simulink library "icc_lib_avg_path1_n1"  (R2018b)
settings: Solver=VariableStepAuto  StartTime=0.0  StopTime=10.0  RelTol=1e-3
undefined symbols (not defined in the file or in its folder): icc_lib_avg_path, path1
libraries: simulink x34, simulink_extras x8, $bdroot x2
(part 3 of 4)

== matlab function icc_lib_avg_path1_n1/freqs ==
  data: cfg2 output; f input
function cfg2 = fcn(f)

% d0=-0.075;
% d1=43.625;
% d2=-0.88;
% d3=-8.65;


d0 = 0;
d1 = 43.5248;
d2= -0.909759259;
d3= -8.636136364;


% VT= -67.6336;
% Vm= -24.1075;
% VR= -28.8921;
% VF= -66.9586;

VT= -67.6339;
Vm= -24.1091;
VR= -28.9894;
VF= -66.9884;

switch f
    % 3.5 cpm
    case 17.15
%         d0 = -0.106346457;
%         d0 = -0.11255;
%         d0 = -0.11847;
        d0 = -0.116;

    % 3.2 cpm
    case 18.75
%         d0 = -0.084943396;
        d0 = -0.09004;
%         d0 = -0.093791667;

    case 20
        d0=-0.0767;
%         d0 = -0.073402174;
    case 20.05
        d0 = -0.073005405;
    case 20.1
       d0 = -0.072612903;
    case 20.15
       d0 = -0.072224599;
    case 20.2
       d0 = -0.071840426;
    case 20.25
       d0 = -0.071460317;
    case 20.3
       d0 = -0.071084211;
    case 20.35
       d0 = -0.070712042;
    case 20.4
       d0 = -0.07034375;
    case 20.45
       d0 = -0.069979275;
    case 20.5
       d0 = -0.069618557;
    case 20.55
       d0 = -0.069261538;
    case 20.6
       d0 = -0.068908163;
    case 20.65
       d0 = -0.068558376;
    case 20.7
       d0 = -0.068212121;
    case 20.75
       d0 = -0.067869347;
    case 20.8
       d0 = -0.06753;
    case 20.85
       d0 = -0.06719403;
    case 20.9
       d0 = -0.066861386;
    case 20.95
       d0 = -0.06653202;
    case 21
       d0 = -0.066205882;
    case 21.05
       d0 = -0.065882927;
    case 21.1
       d0 = -0.065563107;
    case 21.15
       d0 = -0.065246377;
    case 21.2
       d0 = -0.064932692;
    case 21.25
       d0 = -0.06462201;
    case 21.3
       d0 = -0.064314286;
    case 21.35
       d0 = -0.064009479;
    case 21.4
       d0 = -0.063707547;
    case 21.45
       d0 = -0.063408451;
    case 21.5
       d0 = -0.06311215;
    case 21.55
       d0 = -0.062818605;
    case 21.6
       d0 = -0.062527778;
    case 21.65
       d0 = -0.062239631;
    case 21.7
       d0 = -0.061954128;
    case 21.75
       d0 = -0.061671233;
    case 21.8
       d0 = -0.061390909;
    case 21.85
       d0 = -0.061113122;
    case 21.9
       d0 = -0.060837838;
    case 21.95
       d0 = -0.060565022;
    case 22
       d0 = -0.060294643;
    case 22.05
       d0 = -0.060026667;
    case 22.1
       d0 = -0.059761062;
    case 22.15
       d0 = -0.059497797;
    case 22.2
       d0 = -0.059236842;
    case 22.25
       d0 = -0.058978166;
    case 22.3
       d0 = -0.058721739;
    case 22.35
       d0 = -0.058467532;
    case 22.4
       d0 = -0.058215517;
    case 22.45
       d0 = -0.057965665;
    case 22.5
       d0 = -0.057717949;
    case 22.55
       d0 = -0.05747234;
    case 22.6
       d0 = -0.057228814;
    case 22.65
       d0 = -0.056987342;
    case 22.7
       d0 = -0.056747899;
    case 22.75
       d0 = -0.05651046;
    case 22.8
       d0 = -0.056275;
    case 22.85
       d0 = -0.056041494;
    case 22.9
       d0 = -0.055809917;
    case 22.95
       d0 = -0.055580247;
    case 23
       d0 = -0.055352459;
    case 23.05
       d0 = -0.055126531;
    case 23.1
       d0 = -0.054902439;
    case 23.15
       d0 = -0.054680162;
    case 23.2
       d0 = -0.054459677;
    case 23.25
       d0 = -0.054240964;
    case 23.3
       d0 = -0.054024;
    case 23.35
       d0 = -0.053808765;
    case 23.4
       d0 = -0.053595238;
    case 23.45
       d0 = -0.053383399;
    case 23.5
       d0 = -0.053173228;
    case 23.55
       d0 = -0.052964706;
    case 23.6
       d0 = -0.052757812;
    case 23.65
       d0 = -0.052552529;
    case 23.7
       d0 = -0.052348837;
    case 23.75
       d0 = -0.052146718;
    case 23.8
       d0 = -0.051946154;
    case 23.85
       d0 = -0.051747126;
    case 23.9
       d0 = -0.051549618;
    case 23.95
       d0 = -0.051353612;
    case 24
       d0 = -0.051159091;
    case 24.05
       d0 = -0.050966038;
    case 24.1
       d0 = -0.050774436;
    case 24.15
       d0 = -0.05058427;
    case 24.2
       d0 = -0.050395522;
    case 24.25
       d0 = -0.050208178;
    case 24.3
       d0 = -0.050022222;
    case 24.35
       d0 = -0.049837638;
    case 24.4
       d0 = -0.049654412;
    case 24.45
       d0 = -0.049472527;
    case 24.5
       d0 = -0.049291971;
    case 24.55
       d0 = -0.049112727;
    case 24.6
       d0 = -0.048934783;
    case 24.65
       d0 = -0.048758123;
    case 24.7
       d0 = -0.048582734;
    case 24.75
       d0 = -0.048408602;
    case 24.8
       d0 = -0.048235714;
    case 24.85
       d0 = -0.048064057;
    case 24.9
       d0 = -0.047893617;
    case 24.95
       d0 = -0.047724382;
    case 25
       d0 = -0.047556338;
    case 25.05
       d0 = -0.047389474;
    case 25.1
       d0 = -0.047223776;
    case 25.15
       d0 = -0.047059233;
    case 25.2
       d0 = -0.046895833;
    case 25.25
       d0 = -0.046733564;
    case 25.3
       d0 = -0.046572414;
    case 25.35
       d0 = -0.046412371;
    case 25.4
       d0 = -0.046253425;
    case 25.45
       d0 = -0.046095563;
    case 25.5
       d0 = -0.045938776;
    case 25.55
       d0 = -0.045783051;
    case 25.6
       d0 = -0.045628378;
    case 25.65
       d0 = -0.045474747;
    case 25.7
       d0 = -0.045322148;
    case 25.75
       d0 = -0.045170569;
    case 25.8
       d0 = -0.04502;
    case 25.85
       d0 = -0.044870432;
    case 25.9
       d0 = -0.044721854;
    case 25.95
       d0 = -0.044574257;
    case 26
       d0 = -0.044427632;

        
end


cfg2=[d0,d1,d2,d3,VT,Vm,VR,VF];

end

== stateflow chart icc_lib_avg_path1_n1/ICC1/Chart ==
  state wait
    entry:
    du:
    t2=temporalCount (sec);
  state q0
    en:
    q=0
  state q1
    en:
    q=1
    Sense=1;
    exit:
    Sense=0;
  state q3
    en:
    q=3
  state q2
    en:
    q=2
  (default) -> wait : {t2=0;}
  wait -> q0 : [t2>=19.6]{q=0;vreset=-67.6336;reset}
  q0 -> q1 [order 1] : [v<VT]/{vreset=v;Vmax=Vm;d2=d2i;reset}
  q0 -> q1 [order 2] : [gv>VF&&v>VT]{ vreset=gv; Vmax=Vm;d2=d2i;reset}
  q3 -> q0 : [v<VF]{vreset=v; reset}
  q1 -> q2 : [ v >Vmax ]{vreset=v; reset}
  q2 -> q3 : [v<VR]{vreset=v; reset}
  data: v input double; q output; vreset output; gv input double; VT input; Vm input; VR input; VF input; Vmax local; t2 local; d2i input; d2 output; Sense output
  events: reset output EITHER_EDGE_EVENT

== matlab function icc_lib_avg_path1_n1/ICC1/MATLAB Function ==
  data: cfg output
function cfg = fcn()

%d0-o= -0.039651515;
d0= -0.042051515;
d1= 216.5795;
d2= -0.7491129;
d3= -8.890176;
%d3-1= -8.960176;

VT= -67.6;
Vm= -24.3058;
VR= -28.9622;
VF= -66.9799;

cfg=[d0,d1,d2,d3,VT,Vm,VR,VF];

end

== matlab function icc_lib_avg_path1_n1/ICC1/MATLAB Function-freq=22  ==
  data: cfg2 output
function cfg2 = fcn()

%d0-o= -0.039651515;

%d0= -0.042051515;
%d1= 216.5795;
%d2= -0.7491129;
%d3= -8.890176;

%d3-1= -8.960176;

%freq=22
d0=-0.045;
d1=43.5373;
d2=-0.835;
d3=-6.96;


VT= -67.6336;
Vm= -24.1075;
VR= -28.8921;
VF= -66.9586;



cfg2=[d0,d1,d2,d3,VT,Vm,VR,VF];

end

== matlab function icc_lib_avg_path1_n1/freq20 ==
  data: cfg2 output
function cfg2 = fcn()

%d0-o= -0.039651515;

%d0= -0.042051515;
%d1= 216.5795;
%d2= -0.7491129;
%d3= -8.890176;

%d3-1= -8.960176;


d0=-0.075;
d1=43.625;
d2=-0.88;
d3=-8.65;


VT= -67.6336;
Vm= -24.1075;
VR= -28.8921;
VF= -66.9586;



cfg2=[d0,d1,d2,d3,VT,Vm,VR,VF];

end

== stateflow chart icc_lib_avg_path1_n1/Chart1 ==
  state q01
    du:
    t1=temporalCount (sec);
    pulse=-69;
  state q002
    en:m=0;
    du:
    t=temporalCount (sec);
    pulse=-67.6;
  state q001
    en:m=m+1;
    du:
    t=temporalCount (sec);
    pulse=-67.6;
  state state
    en: pulse = -67.6;
  state end
  (default) -> q002 : {m=0; t=0;}
  q001 -> q01 [order 1] : [ t >=5]{ t1=0;}
  q002 -> q001 : [t>=10]{t=0;}
  q01 -> q001 : [t1>=(0.8)]{t=0;}
  q001 -> state [order 2] : [m>6]
  state -> end
  data: m local; t local; t1 local; pulse output

== matlab function icc_lib_avg_path1_n1/ICC /MATLAB Function-freq=26  ==
  data: cfg2 output
function cfg2 = fcn()

%d0-o= -0.039651515;

%d0= -0.042051515;
%d1= 216.5795;
%d2= -0.7491129;
%d3= -8.890176;

%d3-1= -8.960176;

%freq26
d0=-0.053;
d1=39.5735;
d2=-0.8035;
d3=-4.69678;


VT= -67.6336;
Vm= -24.1075;
VR= -28.8921;
VF= -66.9586;



cfg2=[d0,d1,d2,d3,VT,Vm,VR,VF];

end

== stateflow chart icc_lib_avg_path1_n1/ICC-multi/Chart ==
  state wait
    entry:
    du:
    t2=temporalCount (sec);
  state q0
    en:
    q=0
  state q1
    en:
    q=1
  state q3
    en:
    q=3
  state q2
    en:
    q=2
  (default) -> wait : {t2=0;}
  wait -> q0 : [t2>=19.6]{q=0;th=0;vreset=-67.6;reset}
  q0 -> q1 [order 1] : [v<VT]/{vreset=v; th=0; Vmax=Vm;d2=d2i; reset}
  q0 -> q1 [order 2] : [gv>VF&&v>VT]{ vreset=v; th=v-VT/VF-VT; Vmax=func1(th,Vm);d2=func2(th,d2i);reset}
  q3 -> q0 : [v<VF]{vreset=-67; reset}
  q1 -> q2 : [ v >Vmax ]{vreset=v; reset}
  q2 -> q3 : [v<VR]{vreset=v; reset}
  data: vmax function_output double; theta function_input; vm function_input; d2out function_output double; theta function_input; d2in function_input; v input double; q output; vreset output; gv input double; Vmm input; VT input; Vm input; VR input; VF input; th local; Vmax local; t2 local; d2i input; d2 output
  events: reset output EITHER_EDGE_EVENT
  function vmax = func1(theta,vm):
    | function vmax = func1(theta,vm)
    | 
    | m=1;
    | 
    | 
    | vmax1=Vm*exp(-m*th);
    | vmax=-25
  function d2out = func2(theta,d2in):
    | function d2out = func2(theta,d2in)
    | 
    | m=1;
    | 
    | 
    | vmax1=Vm*exp(-m*th);
    | %d2out=-0.5
    | d2out=d2in;

== stateflow chart icc_lib_avg_path1_n1/path/Path ==
  state Relay_cell1
  state Relay_cell2
  state Previous_Direction1
  state Idle
  state Previous_Direction2
  state Wait_cell2
  state Wait_cell1
  state Annihilate
  Wait_cell1 -> Relay_cell1 [order 2] : after(0.1, sec) /
      | {relay1 = 1;
      | last = 1;}
  Wait_cell2 -> Relay_cell2 [order 2] : after(0.1, sec) /
      | {relay2 = 1;
      | last = 2;}
  Relay_cell1 -> Idle : after(0.1, sec) /
      | {relay1 = 0;}
  Relay_cell2 -> Idle : after(0.1, sec) /
      | {relay2 = 0;}
  (default) -> Idle
  Idle -> Previous_Direction2 [order 3] : [mode2 == 2 ...
      | && mode1 ~= 2]
  Previous_Direction2 -> Wait_cell2 [order 2] : [last == 0]
  Idle -> Previous_Direction1 [order 2] : [mode1 == 2 ...
      | && mode2 ~= 2]
  Previous_Direction1 -> Wait_cell1 [order 2] : [last == 0]
  Idle -> Annihilate [order 1] : [mode1 == 2 ...
      | && mode2 == 2]
  Annihilate -> Idle : [mode1 ~= 2 ...
      | && mode2 ~= 2] /
      | {last = 0;}
  Previous_Direction2 -> Wait_cell2 [order 3] : [last == 2]
  Previous_Direction1 -> Wait_cell1 [order 3] : [last == 1]
  Previous_Direction2 -> Wait_cell2 [order 4] : [last == 1 && ...
      | mdelay1 == 0]
  Previous_Direction1 -> Wait_cell1 [order 4] : [last == 2 && ...
      | mdelay2 == 0]
  Wait_cell2 -> Annihilate [order 1] : [mode1 == 2]
  Wait_cell1 -> Annihilate [order 1] : [mode2 == 2]
  Previous_Direction1 -> Annihilate [order 1] : [last == 2 && ...
      | mdelay2 ~= 0]
  Previous_Direction2 -> Annihilate [order 1] : [last == 1 && ...
      | mdelay1 ~= 0]
  data: mode1 input; mdelay1 input; mode2 input; mdelay2 input; relay1 output; relay2 output; last local; cell1_mode_delayed local; cell2_mode_delayed local

== matlab function icc_lib_avg_path1_n1/ICC-multi/MATLAB Function ==
  data: cfg output
function cfg = fcn()

%d0-o= -0.039651515;
d0= -0.042051515;
d1= 216.5795;
d2= -0.7491129;
d3= -8.890176;
%d3-1= -8.960176;

VT= -67.6;
Vm= -24.3058;
VR= -28.9622;
VF= -66.9799;

cfg=[d0,d1,d2,d3,VT,Vm,VR,VF];

end

== matlab function icc_lib_avg_path1_n1/ICC-multi/MATLAB Function-freq=22  ==
  data: cfg2 output
function cfg2 = fcn()

%d0-o= -0.039651515;

%d0= -0.042051515;
%d1= 216.5795;
%d2= -0.7491129;
%d3= -8.890176;

%d3-1= -8.960176;

%freq=22
d0=-0.045;
d1=43.5373;
d2=-0.835;
d3=-6.96;


VT= -67.6336;
Vm= -24.1075;
VR= -28.8921;
VF= -66.9586;



cfg2=[d0,d1,d2,d3,VT,Vm,VR,VF];

end

== matlab function icc_lib_avg_path1_n1/ICC-multi/MATLAB Function-freq=24 ==
  data: cfg2 output
function cfg2 = fcn()

%d0-o= -0.039651515;

%d0= -0.042051515;
%d1= 216.5795;
%d2= -0.7491129;
%d3= -8.890176;

%d3-1= -8.960176;

%freq24
d0=-0.0381;
d1=43.568;
d2=-0.82;
d3=-4.8;


VT= -67.6336;
Vm= -24.1075;
VR= -28.8921;
VF= -66.9586;



cfg2=[d0,d1,d2,d3,VT,Vm,VR,VF];

end

== matlab function icc_lib_avg_path1_n1/ICC-multi/MATLAB Function-freq=26  ==
  data: cfg2 output
function cfg2 = fcn()

%d0-o= -0.039651515;

%d0= -0.042051515;
%d1= 216.5795;
%d2= -0.7491129;
%d3= -8.890176;

%d3-1= -8.960176;

%freq26
d0=-0.053;
d1=39.5735;
d2=-0.8035;
d3=-4.69678;


VT= -67.6336;
Vm= -24.1075;
VR= -28.8921;
VF= -66.9586;



cfg2=[d0,d1,d2,d3,VT,Vm,VR,VF];

end

== matlab function icc_lib_avg_path1_n1/ICC-multi/MATLAB Function-freq=26-o  ==
  data: cfg2 output
function cfg2 = fcn()

%d0-o= -0.039651515;

%d0= -0.042051515;
%d1= 216.5795;
%d2= -0.7491129;
%d3= -8.890176;

%d3-1= -8.960176;

%freq26
d0=-0.053;
d1=39.5735;
d2=-0.8035;
d3=-4.69678;


VT= -67.6336;
Vm= -24.1075;
VR= -28.8921;
VF= -66.9586;



cfg2=[d0,d1,d2,d3,VT,Vm,VR,VF];

end

== matlab function icc_lib_avg_path1_n1/ICC-multi/MATLAB Function1-freq=20  ==
  data: cfg2 output
function cfg2 = fcn()

%d0-o= -0.039651515;

%d0= -0.042051515;
%d1= 216.5795;
%d2= -0.7491129;
%d3= -8.890176;

%d3-1= -8.960176;


d0=-0.075;
d1=43.625;
d2=-0.88;
d3=-8.65;


VT= -67.6336;
Vm= -24.1075;
VR= -28.8921;
VF= -66.9586;



cfg2=[d0,d1,d2,d3,VT,Vm,VR,VF];

end

== matlab function icc_lib_avg_path1_n1/ICC1/MATLAB Function-freq=24 ==
  data: cfg2 output
function cfg2 = fcn()

%d0-o= -0.039651515;

%d0= -0.042051515;
%d1= 216.5795;
%d2= -0.7491129;
%d3= -8.890176;

%d3-1= -8.960176;

%freq24
d0=-0.0381;
d1=43.568;
d2=-0.82;
d3=-4.8;


VT= -67.6336;
Vm= -24.1075;
VR= -28.8921;
VF= -66.9586;



cfg2=[d0,d1,d2,d3,VT,Vm,VR,VF];

end

== matlab function icc_lib_avg_path1_n1/ICC1/MATLAB Function-freq=26  ==
  data: cfg2 output
function cfg2 = fcn()

%d0-o= -0.039651515;

%d0= -0.042051515;
%d1= 216.5795;
%d2= -0.7491129;
%d3= -8.890176;

%d3-1= -8.960176;

%freq26
d0=-0.053;
d1=39.5735;
d2=-0.8035;
d3=-4.69678;


VT= -67.6336;
Vm= -24.1075;
VR= -28.8921;
VF= -66.9586;



cfg2=[d0,d1,d2,d3,VT,Vm,VR,VF];

end

== matlab function icc_lib_avg_path1_n1/ICC1/MATLAB Function-freq=26-o  ==
  data: cfg2 output
function cfg2 = fcn()

%d0-o= -0.039651515;

%d0= -0.042051515;
%d1= 216.5795;
%d2= -0.7491129;
%d3= -8.890176;

%d3-1= -8.960176;

%freq26
d0=-0.053;
d1=39.5735;
d2=-0.8035;
d3=-4.69678;


VT= -67.6336;
Vm= -24.1075;
VR= -28.8921;
VF= -66.9586;



cfg2=[d0,d1,d2,d3,VT,Vm,VR,VF];

end

== matlab function icc_lib_avg_path1_n1/ICC1/MATLAB Function1-freq=20  ==
  data: cfg2 output
function cfg2 = fcn()

%d0-o= -0.039651515;

%d0= -0.042051515;
%d1= 216.5795;
%d2= -0.7491129;
%d3= -8.890176;

%d3-1= -8.960176;


d0=-0.075;
d1=43.625;
d2=-0.88;
d3=-8.65;


VT= -67.6336;
Vm= -24.1075;
VR= -28.8921;
VF= -66.9586;



cfg2=[d0,d1,d2,d3,VT,Vm,VR,VF];

end

== stateflow chart icc_lib_avg_path1_n1/ICC6/Chart ==
  state block
    en:
    q=4
  state wait
    entry:
    du:
    t2=temporalCount (sec);
  state q0
    en:
    q=0
  state q1
    en:
    q=1
    Sense=1
    exit:
    Sense=0
  state q3
    en:
    q=3
  state q2
    en:
    q=2
  wait -> (junction 82) : [t2>=19.6]{q=0;th=0;vreset=-67.6336;reset}
  (junction 82) -> block [order 2] : [b==1]
  (junction 82) -> q0 [order 1] : [b==0]
  (default) -> wait : {t2=0;}
  q0 -> block [order 3] : [b==1]
  block -> q0 : [b==0]
  q0 -> q1 [order 1] : [v<VT]/{vreset=v; th=0; Vmax=Vm;d2=d2i; reset}
  q0 -> q1 [order 2] : [gv>VF&&v>VT]{ vreset=gv; th=v-VT/VF-VT; Vmax=func1(th,Vm);d2=func2(th,d2i);reset}
  q3 -> q0 : [v<VF]{vreset=v; reset}
  q1 -> q2 : [ v >Vmax ]{vreset=v; reset}
  q2 -> q3 : [v<VR]{vreset=v; reset}
  data: vmax function_output double; theta function_input; vm function_input; d2out function_output double; theta function_input; d2in function_input; v input double; q output; vreset output; gv input double; Vmm input; VT input; Vm input; VR input; VF input; th local; Vmax local; t2 local; d2i input; d2 output; b input; Sense output
  events: reset output EITHER_EDGE_EVENT
  function vmax = func1(theta,vm):
    | function vmax = func1(theta,vm)
    | 
    | m=1;
    | 
    | 
    | vmax1=Vm*exp(-m*th);
    | vmax=-25
  function d2out = func2(theta,d2in):
    | function d2out = func2(theta,d2in)
    | 
    | m=1;
    | 
    | 
    | vmax1=Vm*exp(-m*th);
    | %d2out=-0.5
    | d2out=d2in;

== matlab function icc_lib_avg_path1_n1/ICC6/MATLAB Function ==
  data: cfg output
function cfg = fcn()

%d0-o= -0.039651515;
d0= -0.042051515;
d1= 216.5795;
d2= -0.7491129;
d3= -8.890176;
%d3-1= -8.960176;

VT= -67.6;
Vm= -24.3058;
VR= -28.9622;
VF= -66.9799;

cfg=[d0,d1,d2,d3,VT,Vm,VR,VF];

end

== matlab function icc_lib_avg_path1_n1/ICC6/MATLAB Function-freq=22  ==
  data: cfg2 output
function cfg2 = fcn()

%d0-o= -0.039651515;

%d0= -0.042051515;
%d1= 216.5795;
%d2= -0.7491129;
%d3= -8.890176;

%d3-1= -8.960176;

%freq=22
d0=-0.045;
d1=43.5373;
d2=-0.835;
d3=-6.96;


VT= -67.6336;
Vm= -24.1075;
VR= -28.8921;
VF= -66.9586;



cfg2=[d0,d1,d2,d3,VT,Vm,VR,VF];

end

== matlab function icc_lib_avg_path1_n1/ICC6/MATLAB Function-freq=24 ==
  data: cfg2 output
function cfg2 = fcn()

%d0-o= -0.039651515;

%d0= -0.042051515;
%d1= 216.5795;
%d2= -0.7491129;
%d3= -8.890176;

%d3-1= -8.960176;

%freq24
d0=-0.0381;
d1=43.568;
d2=-0.82;
d3=-4.8;


VT= -67.6336;
Vm= -24.1075;
VR= -28.8921;
VF= -66.9586;



cfg2=[d0,d1,d2,d3,VT,Vm,VR,VF];

end

== matlab function icc_lib_avg_path1_n1/ICC6/MATLAB Function-freq=26  ==
  data: cfg2 output
function cfg2 = fcn()

%d0-o= -0.039651515;

%d0= -0.042051515;
%d1= 216.5795;
%d2= -0.7491129;
%d3= -8.890176;

%d3-1= -8.960176;

%freq26
d0=-0.053;
d1=39.5735;
d2=-0.8035;
d3=-4.69678;


VT= -67.6336;
Vm= -24.1075;
VR= -28.8921;
VF= -66.9586;



cfg2=[d0,d1,d2,d3,VT,Vm,VR,VF];

end

== matlab function icc_lib_avg_path1_n1/ICC6/MATLAB Function-freq=26-o  ==
  data: cfg2 output
function cfg2 = fcn()

%d0-o= -0.039651515;

%d0= -0.042051515;
%d1= 216.5795;
%d2= -0.7491129;
%d3= -8.890176;

%d3-1= -8.960176;

%freq26
d0=-0.053;
d1=39.5735;
d2=-0.8035;
d3=-4.69678;


VT= -67.6336;
Vm= -24.1075;
VR= -28.8921;
VF= -66.9586;



cfg2=[d0,d1,d2,d3,VT,Vm,VR,VF];

end

== matlab function icc_lib_avg_path1_n1/ICC6/MATLAB Function1-freq=20  ==
  data: cfg2 output
function cfg2 = fcn()

%d0-o= -0.039651515;

%d0= -0.042051515;
%d1= 216.5795;
%d2= -0.7491129;
%d3= -8.890176;

%d3-1= -8.960176;


d0=-0.075;
d1=43.625;
d2=-0.88;
d3=-8.65;


VT= -67.6336;
Vm= -24.1075;
VR= -28.8921;
VF= -66.9586;



cfg2=[d0,d1,d2,d3,VT,Vm,VR,VF];

end

== stateflow chart icc_lib_avg_path1_n1/ICC5/Chart ==
  state block
    en:
    q=4
  state wait
    entry:
    du:
    t2=temporalCount (sec);
  state q0
    en:
    q=0
  state q1
    en:
    q=1
    Sense=1
    exit:
    Sense=0
  state q3
    en:
    q=3
  state q2
    en:
    q=2
  wait -> (junction 82) : [t2>=19.6]{q=0;th=0;vreset=-67.6336;reset}
  (junction 82) -> block [order 2] : [b==1]
  (junction 82) -> q0 [order 1] : [b==0]
  (default) -> wait : {t2=0;}
  q0 -> block [order 3] : [b==1]
  block -> q0 : [b==0]
  q0 -> q1 [order 1] : [v<VT]/{vreset=v; th=0; Vmax=Vm;d2=d2i; reset}
  q0 -> q1 [order 2] : [gv>VF&&v>VT]{ vreset=gv; th=v-VT/VF-VT; Vmax=func1(th,Vm);d2=func2(th,d2i);reset}
  q3 -> q0 : [v<VF]{vreset=v; reset}
  q1 -> q2 : [ v >Vmax ]{vreset=v; reset}
  q2 -> q3 : [v<VR]{vreset=v; reset}
  data: vmax function_output double; theta function_input; vm function_input; d2out function_output double; theta function_input; d2in function_input; v input double; q output; vreset output; gv input double; Vmm input; VT input; Vm input; VR input; VF input; th local; Vmax local; t2 local; d2i input; d2 output; b input; Sense output
  events: reset output EITHER_EDGE_EVENT
  function vmax = func1(theta,vm):
    | function vmax = func1(theta,vm)
    | 
    | m=1;
    | 
    | 
    | vmax1=Vm*exp(-m*th);
    | vmax=-25
  function d2out = func2(theta,d2in):
    | function d2out = func2(theta,d2in)
    | 
    | m=1;
    | 
    | 
    | vmax1=Vm*exp(-m*th);
    | %d2out=-0.5
    | d2out=d2in;

== matlab function icc_lib_avg_path1_n1/ICC5/MATLAB Function ==
  data: cfg output
function cfg = fcn()

%d0-o= -0.039651515;
d0= -0.042051515;
d1= 216.5795;
d2= -0.7491129;
d3= -8.890176;
%d3-1= -8.960176;

VT= -67.6;
Vm= -24.3058;
VR= -28.9622;
VF= -66.9799;

cfg=[d0,d1,d2,d3,VT,Vm,VR,VF];

end

== matlab function icc_lib_avg_path1_n1/ICC5/MATLAB Function-freq=22  ==
  data: cfg2 output
function cfg2 = fcn()

%d0-o= -0.039651515;

%d0= -0.042051515;
%d1= 216.5795;
%d2= -0.7491129;
%d3= -8.890176;

%d3-1= -8.960176;

%freq=22
d0=-0.045;
d1=43.5373;
d2=-0.835;
d3=-6.96;


VT= -67.6336;
Vm= -24.1075;
VR= -28.8921;
VF= -66.9586;



cfg2=[d0,d1,d2,d3,VT,Vm,VR,VF];

end

== matlab function icc_lib_avg_path1_n1/ICC5/MATLAB Function-freq=24 ==
  data: cfg2 output
function cfg2 = fcn()

%d0-o= -0.039651515;

%d0= -0.042051515;
%d1= 216.5795;
%d2= -0.7491129;
%d3= -8.890176;

%d3-1= -8.960176;

%freq24
d0=-0.0381;
d1=43.568;
d2=-0.82;
d3=-4.8;


VT= -67.6336;
Vm= -24.1075;
VR= -28.8921;
VF= -66.9586;



cfg2=[d0,d1,d2,d3,VT,Vm,VR,VF];

end

== matlab function icc_lib_avg_path1_n1/ICC5/MATLAB Function-freq=26  ==
  data: cfg2 output
function cfg2 = fcn()

%d0-o= -0.039651515;

%d0= -0.042051515;
%d1= 216.5795;
%d2= -0.7491129;
%d3= -8.890176;

%d3-1= -8.960176;

%freq26
d0=-0.053;
d1=39.5735;
d2=-0.8035;
d3=-4.69678;


VT= -67.6336;
Vm= -24.1075;
VR= -28.8921;
VF= -66.9586;



cfg2=[d0,d1,d2,d3,VT,Vm,VR,VF];

end

== matlab function icc_lib_avg_path1_n1/ICC5/MATLAB Function-freq=26-o  ==
  data: cfg2 output
function cfg2 = fcn()

%d0-o= -0.039651515;

%d0= -0.042051515;
%d1= 216.5795;
%d2= -0.7491129;
%d3= -8.890176;

%d3-1= -8.960176;

%freq26
d0=-0.053;
d1=39.5735;
d2=-0.8035;
d3=-4.69678;


VT= -67.6336;
Vm= -24.1075;
VR= -28.8921;
VF= -66.9586;



cfg2=[d0,d1,d2,d3,VT,Vm,VR,VF];

end

== matlab function icc_lib_avg_path1_n1/ICC5/MATLAB Function1-freq=20  ==
  data: cfg2 output
function cfg2 = fcn()

%d0-o= -0.039651515;

%d0= -0.042051515;
%d1= 216.5795;
%d2= -0.7491129;
%d3= -8.890176;

%d3-1= -8.960176;


d0=-0.075;
d1=43.625;
d2=-0.88;
d3=-8.65;


VT= -67.6336;
Vm= -24.1075;
VR= -28.8921;
VF= -66.9586;



cfg2=[d0,d1,d2,d3,VT,Vm,VR,VF];

end

== stateflow chart icc_lib_avg_path1_n1/ICC7/Chart ==
  state block
    en:
    q=4
  state wait
    entry:
    du:
    t2=temporalCount (sec);
  state q0
    en:
    q=0
  state q1
    en:
    q=1
    Sense=1
    exit:
    Sense=0
  state q3
    en:
    q=3
  state q2
    en:
    q=2
  wait -> (junction 82) : [t2>=19.6]{q=0;th=0;vreset=-67.6336;reset}
  (junction 82) -> block [order 2] : [b==1]
  (junction 82) -> q0 [order 1] : [b==0]
  (default) -> wait : {t2=0;}
  q0 -> block [order 3] : [b==1]
  block -> q0 : [b==0]
  q0 -> q1 [order 1] : [v<VT]/{vreset=v; th=0; Vmax=Vm;d2=d2i; reset}
  q0 -> q1 [order 2] : [gv>VF&&v>VT]{ vreset=gv; th=v-VT/VF-VT; Vmax=func1(th,Vm);d2=func2(th,d2i);reset}
  q3 -> q0 : [v<VF]{vreset=v; reset}
  q1 -> q2 : [ v >Vmax ]{vreset=v; reset}
  q2 -> q3 : [v<VR]{vreset=v; reset}
  data: vmax function_output double; theta function_input; vm function_input; d2out function_output double; theta function_input; d2in function_input; v input double; q output; vreset output; gv input double; Vmm input; VT input; Vm input; VR input; VF input; th local; Vmax local; t2 local; d2i input; d2 output; b input; Sense output
  events: reset output EITHER_EDGE_EVENT
  function vmax = func1(theta,vm):
    | function vmax = func1(theta,vm)
    | 
    | m=1;
    | 
    | 
    | vmax1=Vm*exp(-m*th);
    | vmax=-25
  function d2out = func2(theta,d2in):
    | function d2out = func2(theta,d2in)
    | 
    | m=1;
    | 
    | 
    | vmax1=Vm*exp(-m*th);
    | %d2out=-0.5
    | d2out=d2in;

== matlab function icc_lib_avg_path1_n1/ICC7/MATLAB Function ==
  data: cfg output
function cfg = fcn()

%d0-o= -0.039651515;
d0= -0.042051515;
d1= 216.5795;
d2= -0.7491129;
d3= -8.890176;
%d3-1= -8.960176;

VT= -67.6;
Vm= -24.3058;
VR= -28.9622;
VF= -66.9799;

cfg=[d0,d1,d2,d3,VT,Vm,VR,VF];

end

== matlab function icc_lib_avg_path1_n1/ICC7/MATLAB Function-freq=22  ==
  data: cfg2 output
function cfg2 = fcn()

%d0-o= -0.039651515;

%d0= -0.042051515;
%d1= 216.5795;
%d2= -0.7491129;
%d3= -8.890176;

%d3-1= -8.960176;

%freq=22
d0=-0.045;
d1=43.5373;
d2=-0.835;
d3=-6.96;


VT= -67.6336;
Vm= -24.1075;
VR= -28.8921;
VF= -66.9586;



cfg2=[d0,d1,d2,d3,VT,Vm,VR,VF];

end

== stateflow chart icc_lib_avg_path1_n1/Subsystem/Chart ==
  state Pacemaker
    state GRP [parallel]
      settings: executionOrder=1
      state Idle
        du:
        sense=Sense;
      state StartGRP
        du:
        grp=1;
        Tgrp=temporalCount (sec);
      state EndGRP
        en:
        grp=0;
        endGRP=1;
      state Wait
      (default) -> Pacemaker.GRP.Idle : {grp=0;Tgrp=0;endGRP=0;sense=0;}
      Pacemaker.GRP.Idle -> StartGRP [order 1] : [sense==1&&grp==0]{sense=0;}
      StartGRP -> EndGRP : [Tgrp==5]{Tgrp=0;}
      Pacemaker.GRP.Idle -> Pacemaker.GRP.Wait [order 2] : [sense==1&&grp==1]{sense=0;}
      EndGRP -> Pacemaker.GRP.Idle
      Pacemaker.GRP.Wait -> Pacemaker.GRP.Idle
    state LRI [parallel]
      settings: executionOrder=2
      state StartLRI
        en:
        c = c +1;
        du:
        Tlri=temporalCount (sec);
      state EndLRI
        en:
        pace=2;
        du:
        s=Sense
      state Idle
        du:
        s=Sense;
      state wait
      state Wait
      state AfterGRPsense
      (default) -> Pacemaker.LRI.Idle : {Tlri=0;grp=0;endGRP=0;s=0;c=0;}
      StartLRI -> EndLRI [order 1] : [Tlri>func3(c)&&sense==0]{Tlri=0}
      Pacemaker.LRI.Idle -> StartLRI [order 1] : [s==1&&grp==0]{s=0;}
      EndLRI -> StartLRI : [s==1]{pace=0;s=0;endGRP=0}
      Pacemaker.LRI.Wait -> Pacemaker.LRI.Idle
      Pacemaker.LRI.Idle -> Pacemaker.LRI.Wait [order 2] : [s==1&&grp==1]{s=0;}
      AfterGRPsense -> StartLRI
      StartLRI -> AfterGRPsense [order 3] : [endGRP==1&&Tlri<=func3(c)&&sense==1]{Tlri=0;endGRP=0;s=0}
      wait -> StartLRI
      StartLRI -> wait [order 2] : [endGRP==0&&Tlri<=func3(c)&&sense==1]{s=0;}
  (default) -> Pacemaker : {pace=0;}
  data: s local; c local; tlri function_output double; count function_input; pace output; Sense input; Tgrp local; Tlri local; grp local; endGRP local; sense local
  function tlri = func3(count):
    | function tlri = func3(count)
    | 
    | % LRI=19.9;
    | % offset=0.6;
    | 
    | % LRI=19.9-0.2-0.2+0.1;
    | 
    | %pace at s20
    | % offset=0.6+1.6+0.2-0.4;
    | 
    | % pace at s0 (sense and pace at every 20ns, (reveive pace and go upstroke at20n.1s)
    | % LRI = 19.6 making the fixed period as 20s, pace at what expected time use offeset 
    | LRI=19.9-0.2-0.2+0.1; %(LRI = 19.6)
    | offset=0.6+0.2-0.6-0.1; %(offset = 0.1)
    | 
    | % one second delay, i.e.if go upstroke at 20ns, then sense and pace one step advance,i.e set offset as 0 
    | 
    | 
    | %tlri=0;
    | if(count==1)
    |   tlri = LRI+offset;
    | 
    | %elseif(count>1)
    | else
    |   tlri = LRI;
    | 
    | end

== matlab function icc_lib_avg_path1_n1/ICC7/MATLAB Function-freq=24 ==
  data: cfg2 output
function cfg2 = fcn()

%d0-o= -0.039651515;

%d0= -0.042051515;
%d1= 216.5795;
%d2= -0.7491129;
%d3= -8.890176;

%d3-1= -8.960176;

%freq24
d0=-0.0381;
d1=43.568;
d2=-0.82;
d3=-4.8;


VT= -67.6336;
Vm= -24.1075;
VR= -28.8921;
VF= -66.9586;



cfg2=[d0,d1,d2,d3,VT,Vm,VR,VF];

end

== matlab function icc_lib_avg_path1_n1/ICC7/MATLAB Function-freq=26  ==
  data: cfg2 output
function cfg2 = fcn()

%d0-o= -0.039651515;

%d0= -0.042051515;
%d1= 216.5795;
%d2= -0.7491129;
%d3= -8.890176;

%d3-1= -8.960176;

%freq26
d0=-0.053;
d1=39.5735;
d2=-0.8035;
d3=-4.69678;


VT= -67.6336;
Vm= -24.1075;
VR= -28.8921;
VF= -66.9586;



cfg2=[d0,d1,d2,d3,VT,Vm,VR,VF];

end

== matlab function icc_lib_avg_path1_n1/ICC7/MATLAB Function-freq=26-o  ==
  data: cfg2 output
function cfg2 = fcn()

%d0-o= -0.039651515;

%d0= -0.042051515;
%d1= 216.5795;
%d2= -0.7491129;
%d3= -8.890176;

%d3-1= -8.960176;

%freq26
d0=-0.053;
d1=39.5735;
d2=-0.8035;
d3=-4.69678;


VT= -67.6336;
Vm= -24.1075;
VR= -28.8921;
VF= -66.9586;



cfg2=[d0,d1,d2,d3,VT,Vm,VR,VF];

end

== matlab function icc_lib_avg_path1_n1/ICC7/MATLAB Function1-freq=20  ==
  data: cfg2 output
function cfg2 = fcn()

%d0-o= -0.039651515;

%d0= -0.042051515;
%d1= 216.5795;
%d2= -0.7491129;
%d3= -8.890176;

%d3-1= -8.960176;


d0=-0.075;
d1=43.625;
d2=-0.88;
d3=-8.65;


VT= -67.6336;
Vm= -24.1075;
VR= -28.8921;
VF= -66.9586;



cfg2=[d0,d1,d2,d3,VT,Vm,VR,VF];

end

== stateflow chart icc_lib_avg_path1_n1/path1-2/Path ==
  state Relay_cell1
  state Relay_cell2
  state Wait_cell1
  state Idle
  state Wait_cell2
  state Annihilate
  Relay_cell2 -> Idle : after(0.1, sec) /
      | {relay2 = 0;}
  Wait_cell2 -> Relay_cell2 : {relay2 = 1;
      | last = 2;}
  Relay_cell1 -> Idle : after(0.1, sec) /
      | {relay1 = 0;}
  Wait_cell1 -> Relay_cell1 : {relay1 = 1;
      | last = 1;}
  (default) -> Idle
  Idle -> Wait_cell1 [order 2] : [mode1 == 1 ...
      | && mode2 ==0 ]
  Idle -> Wait_cell2 [order 3] : [mode2 == 1 ...
      | && mode1 == 0]
  Idle -> Annihilate [order 1] : [mode1 == 2 ...
      | && mode2 == 2]
  Annihilate -> Idle : [mode1 ~= 2 ...
      | && mode2 ~= 2] /
      | {last = 0;}
  data: mode1 input; mdelay1 input; mode2 input; mdelay2 input; relay1 output; relay2 output; last local =0; cell1_mode_delayed local; cell2_mode_delayed local

== stateflow chart icc_lib_avg_path1_n1/ICC4/Chart ==
  state wait
    entry:
    du:
    t2=temporalCount (sec);
  state q0
    en:
    q=0
  state q1
    en:
    q=1
    Sense=1;
    exit:
    Sense=0;
  state q3
    en:
    q=3
  state q2
    en:
    q=2
  (default) -> wait : {t2=0;}
  wait -> q0 : [t2>=19.6]{q=0;th=0;vreset=-67.6336;reset}
  q0 -> q1 [order 1] : [v<VT]/{vreset=v; th=0; Vmax=Vm;d2=d2i; reset}
  q0 -> q1 [order 2] : [gv>VF&&v>VT]{ vreset=gv; th=v-VT/VF-VT; Vmax=func1(th,Vm);d2=func2(th,d2i);reset}
  q3 -> q0 : [v<VF]{vreset=v; reset}
  q1 -> q2 : [ v >Vmax ]{vreset=v; reset}
  q2 -> q3 : [v<VR]{vreset=v; reset}
  data: vmax function_output double; theta function_input; vm function_input; d2out function_output double; theta function_input; d2in function_input; v input double; q output; vreset output; gv input double; Vmm input; VT input; Vm input; VR input; VF input; th local; Vmax local; t2 local; d2i input; d2 output; Sense output
  events: reset output EITHER_EDGE_EVENT
  function vmax = func1(theta,vm):
    | function vmax = func1(theta,vm)
    | 
    | m=1;
    | 
    | 
    | vmax1=Vm*exp(-m*th);
    | vmax=-25
  function d2out = func2(theta,d2in):
    | function d2out = func2(theta,d2in)
    | 
    | m=1;
    | 
    | 
    | vmax1=Vm*exp(-m*th);
    | %d2out=-0.5
    | d2out=d2in;

== matlab function icc_lib_avg_path1_n1/ICC4/MATLAB Function ==
  data: cfg output
function cfg = fcn()

%d0-o= -0.039651515;
d0= -0.042051515;
d1= 216.5795;
d2= -0.7491129;
d3= -8.890176;
%d3-1= -8.960176;

VT= -67.6;
Vm= -24.3058;
VR= -28.9622;
VF= -66.9799;

cfg=[d0,d1,d2,d3,VT,Vm,VR,VF];

end

== matlab function icc_lib_avg_path1_n1/ICC4/MATLAB Function-freq=22  ==
  data: cfg2 output
function cfg2 = fcn()

%d0-o= -0.039651515;

%d0= -0.042051515;
%d1= 216.5795;
%d2= -0.7491129;
%d3= -8.890176;

%d3-1= -8.960176;

%freq=22
d0=-0.045;
d1=43.5373;
d2=-0.835;
d3=-6.96;


VT= -67.6336;
Vm= -24.1075;
VR= -28.8921;
VF= -66.9586;



cfg2=[d0,d1,d2,d3,VT,Vm,VR,VF];

end

== matlab function icc_lib_avg_path1_n1/ICC4/MATLAB Function-freq=24 ==
  data: cfg2 output
function cfg2 = fcn()

%d0-o= -0.039651515;

%d0= -0.042051515;
%d1= 216.5795;
%d2= -0.7491129;
%d3= -8.890176;

%d3-1= -8.960176;

%freq24
d0=-0.0381;
d1=43.568;
d2=-0.82;
d3=-4.8;


VT= -67.6336;
Vm= -24.1075;
VR= -28.8921;
VF= -66.9586;



cfg2=[d0,d1,d2,d3,VT,Vm,VR,VF];

end

== matlab function icc_lib_avg_path1_n1/ICC4/MATLAB Function-freq=26  ==
  data: cfg2 output
function cfg2 = fcn()

%d0-o= -0.039651515;

%d0= -0.042051515;
%d1= 216.5795;
%d2= -0.7491129;
%d3= -8.890176;

%d3-1= -8.960176;

%freq26
d0=-0.053;
d1=39.5735;
d2=-0.8035;
d3=-4.69678;


VT= -67.6336;
Vm= -24.1075;
VR= -28.8921;
VF= -66.9586;



cfg2=[d0,d1,d2,d3,VT,Vm,VR,VF];

end

== matlab function icc_lib_avg_path1_n1/ICC4/MATLAB Function-freq=26-o  ==
  data: cfg2 output
function cfg2 = fcn()

%d0-o= -0.039651515;

%d0= -0.042051515;
%d1= 216.5795;
%d2= -0.7491129;
%d3= -8.890176;

%d3-1= -8.960176;

%freq26
d0=-0.053;
d1=39.5735;
d2=-0.8035;
d3=-4.69678;


VT= -67.6336;
Vm= -24.1075;
VR= -28.8921;
VF= -66.9586;



cfg2=[d0,d1,d2,d3,VT,Vm,VR,VF];

end

== matlab function icc_lib_avg_path1_n1/ICC4/MATLAB Function1-freq=20  ==
  data: cfg2 output
function cfg2 = fcn()

%d0-o= -0.039651515;

%d0= -0.042051515;
%d1= 216.5795;
%d2= -0.7491129;
%d3= -8.890176;

%d3-1= -8.960176;


d0=-0.075;
d1=43.625;
d2=-0.88;
d3=-8.65;


VT= -67.6336;
Vm= -24.1075;
VR= -28.8921;
VF= -66.9586;



cfg2=[d0,d1,d2,d3,VT,Vm,VR,VF];

end

== stateflow chart icc_lib_avg_path1_n1/EGM/Path2 ==
  state EGM1
    state De_wave_i [parallel]
      settings: executionOrder=1
      state Idle
        en:
        egm_i = 0;
      state Active
        du:
        egm_i  = EGM(cvi,xi,yi,xj,yj,t1,0,20,1,C);
      EGM1.De_wave_i.Idle -> EGM1.De_wave_i.Active : [t1~=0]
      (default) -> EGM1.De_wave_i.Idle
      EGM1.De_wave_i.Active -> EGM1.De_wave_i.Idle : [t1==0]
    state De_wave_j [parallel]
      settings: executionOrder=2
      state Idle
        en:
        egm_j = 0;
      state Active
        du:
        egm_j = EGM(cvj,xj,yj,xi,yi,t2,0,20,1,C);
      EGM1.De_wave_j.Idle -> EGM1.De_wave_j.Active : [t2~=0]
      (default) -> EGM1.De_wave_j.Idle
      EGM1.De_wave_j.Active -> EGM1.De_wave_j.Idle : [t2==0]
  (default) -> EGM1
  data: cv1in function_input; x1in function_input; y1in function_input; x2in function_input; y2in function_input; t1in function_input; xe function_input; ye function_input; ze function_input; Cin function_input; Potential_d function_output; xi input; yi input; xj input; yj input; cvi input; cvj input; t1 input; t2 input; C input; egm_i output; egm_j output
  function Potential_d = EGM(cv1in,x1in,y1in,x2in,y2in,t1in,xe,ye,ze,Cin):
    | function Potential_d = EGM(cv1in,x1in,y1in,x2in,y2in,t1in,xe,ye,ze,Cin)
    |     %#codegen
    |     % % The distance (mm) between the electrodes and the activation in z
    |     % direction
    |     % Compute theta2: the angle between (x1,y1)-->(x2,y2) and x axis;
    |     cos_theta2=(x2in-x1in)/sqrt((x2in-x1in)^2+(y2in-y1in)^2);
    |     sin_theta2=(y1in-y2in)/sqrt((x2in-x1in)^2+(y2in-y1in)^2);
    |     if cos_theta2~=0
    |     tan_theta2=(y1in-y2in)/(x2in-x1in);
    |     else
    |      tan_theta2=0;   
    |     end
    |     
    | %     N=length(electrodein)-4; % The number of (x,y,z) of total micro electrodes;
    | %     
    | %     vtip=electrodein(length(electrodein)); % The number of micro electrodes of the ventricular tip part;
    | %     vring=electrodein(length(electrodein)-1); % The number of micro electrodes of the ventricular ring part;
    | %     atip=electrodein(length(electrodein)-2); % The number of micro electrodes of the atrial tip part;
    | %     aring=electrodein(length(electrodein)-3); % The number of micro electrodes of the atrial ring part;
    | %     Potential_d=zeros(1,4); % To store the EGM sensed by atrial ring, tip, ventricular ring and tip part;
    | %     p=zeros(1,N/3); % To store the signals sensed by all the micro electrodes;
    | 
    |     L=1; % weighting factor of the longitudinal dipole
    |     T=0.1; % weighting factor of the transversal dipole
    |     % Only when the path is active, can the cells contribute to the EGM
    | %     m=0;
    | %     for j=1:3:(N-2)
    |     % The location of the micro electrode
    | %     x3=electrodein(j);
    | %     y3=electrodein(j+1);
    | %     zin=electrodein(j+2);
    |     % The closest point to the micro electrode
    |     if cos_theta2~=0
    |         y4=(y2in+tan_theta2*(x2in-xe+tan_theta2*ye))/(1+tan_theta2^2);
    |         x4=tan_theta2*y4-tan_theta2*ye+xe;
    |     else
    |         y4=ye;
    |         x4=x1in;
    |     end
    |     d=sqrt((xe-x4)^2+(ye-y4)^2+ze^2);
    | 
    |     x11=x1in+cv1in*t1in*cos_theta2; % the dipole position
    |     y11=y1in-cv1in*t1in*sin_theta2;
    |     % Compute theta1: the angle between (x11,y11)-->(x3,y3) and x axis;
    |     if xe==x11 && ye==y11
    |      cos_theta1=0;
    |      sin_theta1=0;
    |     else
    |         cos_theta1=(xe-x11)/sqrt((xe-x11)^2+(ye-y11)^2);
    |         sin_theta1=(ye-y11)/sqrt((xe-x11)^2+(ye-y11)^2);
    |     end
    |     % alfa=theta1+theta2, the angle between (x11,y11)-->(x3,y3) and (x11,y11)-->(x2,y2)
    |     cos_alfa = cos_theta1*cos_theta2 - sin_theta1*sin_theta2;
    | 
    |     h1=sqrt((x4-x11)^2+(y4-y11)^2)*sign(cos_alfa); % the distance between the dipole and (x4,y4), when the dipole is approaching, h1>0;
    |     r1=sqrt((d^2+h1^2)); % the distance between the dipole and the micro electrode;
    |     EGML1=L*h1/(r1^3);
    |     EGMT1=(-1)*T*d/(r1^3);
    |     EGMall=EGML1+EGMT1;
    | %     m=m+1;
    | %     p(m) =EGMall*Cin;
    |     Potential_d=EGMall*Cin;
    | %     end
    | %     s=1;
    | %     e=aring;
    | %     Potential_d(1)=sum(p(s:e));
    | %     s=e+1;
    | %     e=s+atip-1;
    | %     Potential_d(2)=sum(p(s:e));
    | %     s=e+1;
    | %     e=s+vring-1;
    | %     Potential_d(3)=sum(p(s:e));
    | %     s=e+1;
    | %     e=s+vtip-1;
    | %     Potential_d(4)=sum(p(s:e));
    | 
    | end

== stateflow chart icc_lib_avg_path1_n1/path_EGM/Path ==
  state Relay_cell1
  state Relay_cell2
  state Wait_cell1
    du:
    t1=temporalCount(sec);
    ex:
    t1=0;
  state Idle
  state Wait_cell2
    du:
    t2=temporalCount(sec);
    ex:
    t2=0;
  state Annihilate
  Relay_cell2 -> Idle : after(0.1, sec) /
      | {relay2 = 0;}
  Wait_cell2 -> Relay_cell2 : [t2>=1]{relay2 = 1;
      | last = 2;}
  Relay_cell1 -> Idle : after(0.1, sec) /
      | {relay1 = 0;}
  Wait_cell1 -> Relay_cell1 : [t1>=1]{relay1 = 1;
      | last = 1;}
  (default) -> Idle : {t1=0; t2=0;}
  Idle -> Wait_cell1 [order 2] : [mode1 == 1 ...
      | && mode2 ==0 ]
  Idle -> Wait_cell2 [order 3] : [mode2 == 1 ...
      | && mode1 == 0]
  Idle -> Annihilate [order 1] : [mode1 == 2 ...
      | && mode2 == 2]
  Annihilate -> Idle : [mode1 ~= 2 ...
      | && mode2 ~= 2] /
      | {last = 0;}
  data: mode1 input; mdelay1 input; mode2 input; mdelay2 input; relay1 output; relay2 output; last local =0; cell1_mode_delayed local; cell2_mode_delayed local; t1 output; t2 output

== matlab function icc_lib_avg_path1_n1/cfg ==
  data: cfg2 output; f input; x input; y input
function cfg2 = fcn(f,x,y)


d0 = 0;
d1 = 43.5248;
d2= -0.909759259;
d3= -8.636136364;


VT= -67.6339;
Vm= -24.1091;
VR= -28.9894;
VF= -66.9884;

switch f

    case 20
       d0 = -0.069979275;

    case 21.5
       d0 = -0.060294643;

    case 23
       d0 = -0.052964706;

    case 24.5
       d0 = -0.047223776;

    case 26
       d0 = -0.042471698;
        
end


cfg2=[d0,d1,d2,d3,VT,Vm,VR,VF,x,y];

end

== stateflow chart icc_lib_avg_path1_n1/ICC1_egm/Chart ==
  state wait
    entry:
    du:
    t2=temporalCount (sec);
  state q0
    en:
    q=0
  state q1
    en:
    q=1
    Sense=1;
    exit:
    Sense=0;
  state q3
    en:
    q=3
  state q2
    en:
    q=2
  (default) -> wait : {t2=0;}
  wait -> q0 : [t2>=19.999]{q=0;vreset=-67.6336;reset}
  q0 -> q1 [order 1] : [v<VT]/{vreset=v;Vmax=Vm;d2=d2i;reset}
  q0 -> q1 [order 2] : [gv>VF&&v>VT]{ vreset=v; Vmax=Vm;d2=d2i;reset}
  q3 -> q0 : [v<VF]{vreset=v; reset}
  q1 -> q2 : [ v >Vmax ]{vreset=v; reset}
  q2 -> q3 : [v<VR]{vreset=v; reset}
  data: v input double; q output; vreset output; gv input double; VT input; Vm input; VR input; VF input; Vmax local; t2 local; d2i input; d2 output; Sense output
  events: reset output EITHER_EDGE_EVENT

== matlab function icc_lib_avg_path1_n1/ICC1_egm/MATLAB Function ==
  data: cfg output
function cfg = fcn()

%d0-o= -0.039651515;
d0= -0.042051515;
d1= 216.5795;
d2= -0.7491129;
d3= -8.890176;
%d3-1= -8.960176;

VT= -67.6;
Vm= -24.3058;
VR= -28.9622;
VF= -66.9799;

cfg=[d0,d1,d2,d3,VT,Vm,VR,VF];

end

== matlab function icc_lib_avg_path1_n1/ICC1_egm/MATLAB Function-freq=22  ==
  data: cfg2 output
function cfg2 = fcn()

%d0-o= -0.039651515;

%d0= -0.042051515;
%d1= 216.5795;
%d2= -0.7491129;
%d3= -8.890176;

%d3-1= -8.960176;

%freq=22
d0=-0.045;
d1=43.5373;
d2=-0.835;
d3=-6.96;


VT= -67.6336;
Vm= -24.1075;
VR= -28.8921;
VF= -66.9586;



cfg2=[d0,d1,d2,d3,VT,Vm,VR,VF];

end

== matlab function icc_lib_avg_path1_n1/ICC1_egm/MATLAB Function-freq=24 ==
  data: cfg2 output
function cfg2 = fcn()

%d0-o= -0.039651515;

%d0= -0.042051515;
%d1= 216.5795;
%d2= -0.7491129;
%d3= -8.890176;

%d3-1= -8.960176;

%freq24
d0=-0.0381;
d1=43.568;
d2=-0.82;
d3=-4.8;


VT= -67.6336;
Vm= -24.1075;
VR= -28.8921;
VF= -66.9586;



cfg2=[d0,d1,d2,d3,VT,Vm,VR,VF];

end

== matlab function icc_lib_avg_path1_n1/ICC1_egm/MATLAB Function-freq=26  ==
  data: cfg2 output
function cfg2 = fcn()

%d0-o= -0.039651515;

%d0= -0.042051515;
%d1= 216.5795;
%d2= -0.7491129;
%d3= -8.890176;

%d3-1= -8.960176;

%freq26
d0=-0.053;
d1=39.5735;
d2=-0.8035;
d3=-4.69678;


VT= -67.6336;
Vm= -24.1075;
VR= -28.8921;
VF= -66.9586;



cfg2=[d0,d1,d2,d3,VT,Vm,VR,VF];

end

== matlab function icc_lib_avg_path1_n1/ICC1_egm/MATLAB Function-freq=26-o  ==
  data: cfg2 output
function cfg2 = fcn()

%d0-o= -0.039651515;

%d0= -0.042051515;
%d1= 216.5795;
%d2= -0.7491129;
%d3= -8.890176;

%d3-1= -8.960176;

%freq26
d0=-0.053;
d1=39.5735;
d2=-0.8035;
d3=-4.69678;


VT= -67.6336;
Vm= -24.1075;
VR= -28.8921;
VF= -66.9586;



cfg2=[d0,d1,d2,d3,VT,Vm,VR,VF];

end

== matlab function icc_lib_avg_path1_n1/ICC1_egm/MATLAB Function1-freq=20  ==
  data: cfg2 output
function cfg2 = fcn()

%d0-o= -0.039651515;

%d0= -0.042051515;
%d1= 216.5795;
%d2= -0.7491129;
%d3= -8.890176;

%d3-1= -8.960176;


d0=-0.075;
d1=43.625;
d2=-0.88;
d3=-8.65;


VT= -67.6336;
Vm= -24.1075;
VR= -28.8921;
VF= -66.9586;



cfg2=[d0,d1,d2,d3,VT,Vm,VR,VF];

end

== stateflow chart icc_lib_avg_path1_n1/ICC4_egm/Chart ==
  state wait
    entry:
    du:
    t2=temporalCount (sec);
  state q0
    en:
    q=0
  state q1
    en:
    q=1
    Sense=1;
    exit:
    Sense=0;
  state q3
    en:
    q=3
  state q2
    en:
    q=2
  (default) -> wait : {t2=0;}
  wait -> q0 : [t2>=19.999]{q=0;th=0;vreset=-67.6336;reset}
  q0 -> q1 [order 1] : [v<VT]/{vreset=v; th=0; Vmax=Vm;d2=d2i; reset}
  q0 -> q1 [order 2] : [gv>VF&&v>VT]{ vreset=v; th=v-VT/VF-VT; Vmax=func1(th,Vm);d2=func2(th,d2i);reset}
  q3 -> q0 : [v<VF]{vreset=v; reset}
  q1 -> q2 : [ v >Vmax ]{vreset=v; reset}
  q2 -> q3 : [v<VR]{vreset=v; reset}
  data: vmax function_output double; theta function_input; vm function_input; d2out function_output double; theta function_input; d2in function_input; v input double; q output; vreset output; gv input double; Vmm input; VT input; Vm input; VR input; VF input; th local; Vmax local; t2 local; d2i input; d2 output; Sense output
  events: reset output EITHER_EDGE_EVENT
  function vmax = func1(theta,vm):
    | function vmax = func1(theta,vm)
    | 
    | m=1;
    | 
    | 
    | vmax1=Vm*exp(-m*th);
    | vmax=-25
  function d2out = func2(theta,d2in):
    | function d2out = func2(theta,d2in)
    | 
    | m=1;
    | 
    | 
    | vmax1=Vm*exp(-m*th);
    | %d2out=-0.5
    | d2out=d2in;

== matlab function icc_lib_avg_path1_n1/ICC4_egm/MATLAB Function ==
  data: cfg output
function cfg = fcn()

%d0-o= -0.039651515;
d0= -0.042051515;
d1= 216.5795;
d2= -0.7491129;
d3= -8.890176;
%d3-1= -8.960176;

VT= -67.6;
Vm= -24.3058;
VR= -28.9622;
VF= -66.9799;

cfg=[d0,d1,d2,d3,VT,Vm,VR,VF];

end

== matlab function icc_lib_avg_path1_n1/ICC4_egm/MATLAB Function-freq=22  ==
  data: cfg2 output
function cfg2 = fcn()

%d0-o= -0.039651515;

%d0= -0.042051515;
%d1= 216.5795;
%d2= -0.7491129;
%d3= -8.890176;

%d3-1= -8.960176;

%freq=22
d0=-0.045;
d1=43.5373;
d2=-0.835;
d3=-6.96;


VT= -67.6336;
Vm= -24.1075;
VR= -28.8921;
VF= -66.9586;



cfg2=[d0,d1,d2,d3,VT,Vm,VR,VF];

end

== matlab function icc_lib_avg_path1_n1/ICC4_egm/MATLAB Function-freq=24 ==
  data: cfg2 output
function cfg2 = fcn()

%d0-o= -0.039651515;

%d0= -0.042051515;
%d1= 216.5795;
%d2= -0.7491129;
%d3= -8.890176;

%d3-1= -8.960176;

%freq24
d0=-0.0381;
d1=43.568;
d2=-0.82;
d3=-4.8;


VT= -67.6336;
Vm= -24.1075;
VR= -28.8921;
VF= -66.9586;



cfg2=[d0,d1,d2,d3,VT,Vm,VR,VF];

end

== matlab function icc_lib_avg_path1_n1/ICC4_egm/MATLAB Function-freq=26  ==
  data: cfg2 output
function cfg2 = fcn()

%d0-o= -0.039651515;

%d0= -0.042051515;
%d1= 216.5795;
%d2= -0.7491129;
%d3= -8.890176;

%d3-1= -8.960176;

%freq26
d0=-0.053;
d1=39.5735;
d2=-0.8035;
d3=-4.69678;


VT= -67.6336;
Vm= -24.1075;
VR= -28.8921;
VF= -66.9586;



cfg2=[d0,d1,d2,d3,VT,Vm,VR,VF];

end

== matlab function icc_lib_avg_path1_n1/ICC4_egm/MATLAB Function-freq=26-o  ==
  data: cfg2 output
function cfg2 = fcn()

%d0-o= -0.039651515;

%d0= -0.042051515;
%d1= 216.5795;
%d2= -0.7491129;
%d3= -8.890176;

%d3-1= -8.960176;

%freq26
d0=-0.053;
d1=39.5735;
d2=-0.8035;
d3=-4.69678;


VT= -67.6336;
Vm= -24.1075;
VR= -28.8921;
VF= -66.9586;



cfg2=[d0,d1,d2,d3,VT,Vm,VR,VF];

end

== matlab function icc_lib_avg_path1_n1/ICC4_egm/MATLAB Function1-freq=20  ==
  data: cfg2 output
function cfg2 = fcn()

%d0-o= -0.039651515;

%d0= -0.042051515;
%d1= 216.5795;
%d2= -0.7491129;
%d3= -8.890176;

%d3-1= -8.960176;


d0=-0.075;
d1=43.625;
d2=-0.88;
d3=-8.65;


VT= -67.6336;
Vm= -24.1075;
VR= -28.8921;
VF= -66.9586;



cfg2=[d0,d1,d2,d3,VT,Vm,VR,VF];

end

== stateflow chart icc_lib_avg_path1_n1/ICC5_egm/Chart ==
  state block
    en:
    q=4
  state wait
    entry:
    du:
    t2=temporalCount (sec);
  state q0
    en:
    q=0
  state q1
    en:
    q=1
    Sense=1
    exit:
    Sense=0
  state q3
    en:
    q=3
  state q2
    en:
    q=2
  wait -> (junction 82) : [t2>=19.999]{q=0;th=0;vreset=-67.6336;reset}
  (junction 82) -> block [order 2] : [b==1]
  (junction 82) -> q0 [order 1] : [b==0]
  (default) -> wait : {t2=0;}
  q0 -> block [order 3] : [b==1]
  block -> q0 : [b==0]
  q0 -> q1 [order 1] : [v<VT]/{vreset=v; th=0; Vmax=Vm;d2=d2i; reset}
  q0 -> q1 [order 2] : [gv>VF&&v>VT]{ vreset=v; th=v-VT/VF-VT; Vmax=func1(th,Vm);d2=func2(th,d2i);reset}
  q3 -> q0 : [v<VF]{vreset=v; reset}
  q1 -> q2 : [ v >Vmax ]{vreset=v; reset}
  q2 -> q3 : [v<VR]{vreset=v; reset}
  data: vmax function_output double; theta function_input; vm function_input; d2out function_output double; theta function_input; d2in function_input; v input double; q output; vreset output; gv input double; Vmm input; VT input; Vm input; VR input; VF input; th local; Vmax local; t2 local; d2i input; d2 output; b input; Sense output
  events: reset output EITHER_EDGE_EVENT
  function vmax = func1(theta,vm):
    | function vmax = func1(theta,vm)
    | 
    | m=1;
    | 
    | 
    | vmax1=Vm*exp(-m*th);
    | vmax=-25
  function d2out = func2(theta,d2in):
    | function d2out = func2(theta,d2in)
    | 
    | m=1;
    | 
    | 
    | vmax1=Vm*exp(-m*th);
    | %d2out=-0.5
    | d2out=d2in;

== matlab function icc_lib_avg_path1_n1/ICC5_egm/MATLAB Function ==
  data: cfg output
function cfg = fcn()

%d0-o= -0.039651515;
d0= -0.042051515;
d1= 216.5795;
d2= -0.7491129;
d3= -8.890176;
%d3-1= -8.960176;

VT= -67.6;
Vm= -24.3058;
VR= -28.9622;
VF= -66.9799;

cfg=[d0,d1,d2,d3,VT,Vm,VR,VF];

end

== matlab function icc_lib_avg_path1_n1/ICC5_egm/MATLAB Function-freq=22  ==
  data: cfg2 output
function cfg2 = fcn()

%d0-o= -0.039651515;

%d0= -0.042051515;
%d1= 216.5795;
%d2= -0.7491129;
%d3= -8.890176;

%d3-1= -8.960176;

%freq=22
d0=-0.045;
d1=43.5373;
d2=-0.835;
d3=-6.96;


VT= -67.6336;
Vm= -24.1075;
VR= -28.8921;
VF= -66.9586;



cfg2=[d0,d1,d2,d3,VT,Vm,VR,VF];

end

== matlab function icc_lib_avg_path1_n1/ICC5_egm/MATLAB Function-freq=24 ==
  data: cfg2 output
function cfg2 = fcn()

%d0-o= -0.039651515;

%d0= -0.042051515;
%d1= 216.5795;
%d2= -0.7491129;
%d3= -8.890176;

%d3-1= -8.960176;

%freq24
d0=-0.0381;
d1=43.568;
d2=-0.82;
d3=-4.8;


VT= -67.6336;
Vm= -24.1075;
VR= -28.8921;
VF= -66.9586;



cfg2=[d0,d1,d2,d3,VT,Vm,VR,VF];

end

== matlab function icc_lib_avg_path1_n1/ICC5_egm/MATLAB Function-freq=26  ==
  data: cfg2 output
function cfg2 = fcn()

%d0-o= -0.039651515;

%d0= -0.042051515;
%d1= 216.5795;
%d2= -0.7491129;
%d3= -8.890176;

%d3-1= -8.960176;

%freq26
d0=-0.053;
d1=39.5735;
d2=-0.8035;
d3=-4.69678;


VT= -67.6336;
Vm= -24.1075;
VR= -28.8921;
VF= -66.9586;



cfg2=[d0,d1,d2,d3,VT,Vm,VR,VF];

end

== matlab function icc_lib_avg_path1_n1/ICC5_egm/MATLAB Function-freq=26-o  ==
  data: cfg2 output
function cfg2 = fcn()

%d0-o= -0.039651515;

%d0= -0.042051515;
%d1= 216.5795;
%d2= -0.7491129;
%d3= -8.890176;

%d3-1= -8.960176;

%freq26
d0=-0.053;
d1=39.5735;
d2=-0.8035;
d3=-4.69678;


VT= -67.6336;
Vm= -24.1075;
VR= -28.8921;
VF= -66.9586;



cfg2=[d0,d1,d2,d3,VT,Vm,VR,VF];

end

== matlab function icc_lib_avg_path1_n1/ICC5_egm/MATLAB Function1-freq=20  ==
  data: cfg2 output
function cfg2 = fcn()

%d0-o= -0.039651515;

%d0= -0.042051515;
%d1= 216.5795;
%d2= -0.7491129;
%d3= -8.890176;

%d3-1= -8.960176;


d0=-0.075;
d1=43.625;
d2=-0.88;
d3=-8.65;


VT= -67.6336;
Vm= -24.1075;
VR= -28.8921;
VF= -66.9586;



cfg2=[d0,d1,d2,d3,VT,Vm,VR,VF];

end
